simulink model "stm32eth"  (R2024a)
settings: Solver=FixedStepAuto  StartTime=0.0  StopTime=10  FixedStep=1/400  RelTol=1e-3  EnableMultiTasking=on
model workspace (MAT data in the model file):
  samp_time = 0.0025
libraries: stm32f4xxblockslib x6, spsTriangleGeneratorLib x1
settings Model: STM32="{\"DigitalPortWrite\":[{\"ID\":\"stm32eth:46\"},{\"ID\":\"stm32eth:45\"},{\"ID\":\"stm32eth:44\"},{\"ID\":\"stm32eth:43\"},{\"ID\":\"stm32eth:42\"},{\"ID\":\"stm32eth:41\"}]}"  Creator=Konstantin  LastModifiedBy=Konstantin
settings OptimizationCC: EnhancedBackFolding=on  PassReuseOutputArgsAs=Individual arguments  ZeroExternalMemoryAtStartup=off  ZeroInternalMemoryAtStartup=off  MaxStackSize=64  OptimizeBlockOrder=speed  DifferentSizesBufferReuse=on  OptimizationCustomize=off  EfficientTunableParamExpr=on
settings DebuggingCC: ParameterTunabilityLossMsg=error
settings HardwareCC: ProdBitPerPointer=32  ProdBitPerSizeT=32  ProdBitPerPtrDiffT=32  ProdLargestAtomicInteger=Long  ProdLargestAtomicFloat=Double  ProdWordSize=32  ProdLongLongMode=on  ProdHWDeviceType=ARM Compatible->ARM Cortex-M
settings SFSimCC: MATLABDynamicMemAlloc=off
settings RTWCC: Description=Embedded Coder  SystemTargetFile=ert.tlc  HardwareBoard=STM32G4xx Based  TemplateMakefile=ert_default_tmf  Toolchain=GNU Tools for ARM Embedded Processors
settings CodeAppCC: ForceParamTrailComments=on  IgnoreCustomStorageClasses=off  OperatorAnnotations=on  SimulinkDataObjDesc=on  SFDataObjDesc=on  InsertBlockDesc=on
settings ERTTargetCC: TargetLangStandard=C99 (ISO)  CodeReplacementLibrary=ARM Cortex-M  ExtModeTransport=3  ExtModeStaticAlloc=on  ExtModeStaticAllocSize=2048  ExtModeMexFile=ext_xcp  ExtModeIntrfLevel=Level2 - Open

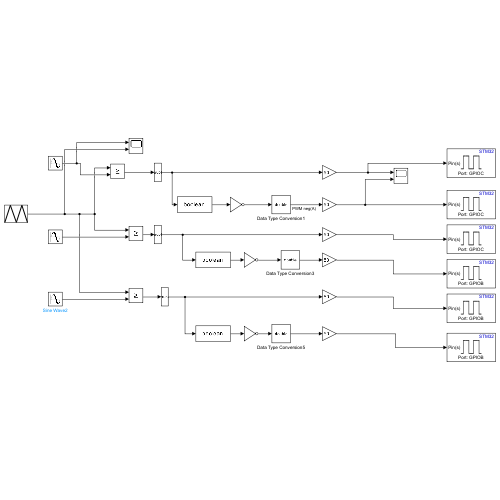
[thumbnail: Simulink's stored preview of the top-level diagram]
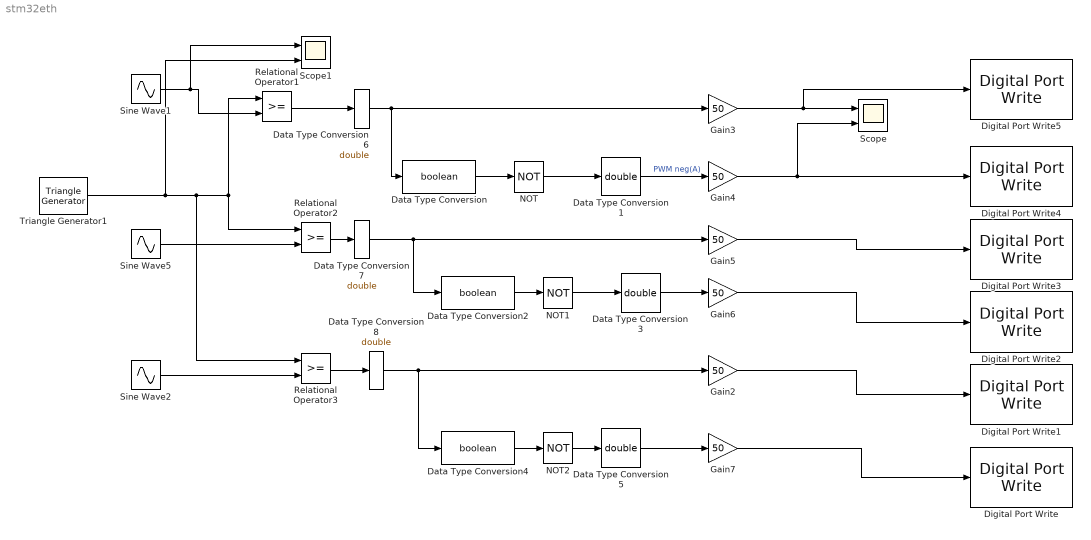
== system stm32eth ==
  Data Type Conversion : DataTypeConversion  OutDataTypeStr=boolean  SaturateOnIntegerOverflow=off  RndMeth=Floor
  Data Type Conversion1 : DataTypeConversion  OutDataTypeStr=double  RndMeth=Nearest  SaturateOnIntegerOverflow=off
  Data Type Conversion2 : DataTypeConversion  OutDataTypeStr=boolean  SaturateOnIntegerOverflow=off  RndMeth=Floor
  Data Type Conversion3 : DataTypeConversion  OutDataTypeStr=double  RndMeth=Nearest  SaturateOnIntegerOverflow=off
  Data Type Conversion4 : DataTypeConversion  OutDataTypeStr=boolean  SaturateOnIntegerOverflow=off  RndMeth=Floor
  Data Type Conversion5 : DataTypeConversion  OutDataTypeStr=double  RndMeth=Nearest  SaturateOnIntegerOverflow=off
  Data Type Conversion6 : DataTypeConversion  OutDataTypeStr=double  SaturateOnIntegerOverflow=off  RndMeth=Floor
  Data Type Conversion7 : DataTypeConversion  OutDataTypeStr=double  SaturateOnIntegerOverflow=off  RndMeth=Floor
  Data Type Conversion8 : DataTypeConversion  OutDataTypeStr=double  SaturateOnIntegerOverflow=off  RndMeth=Floor
  Digital Port Write : stm32f4xxblockslib/Digital Port Write  PortName=GPIOB  PinNumber=[5]  ReadOperation=off  IOAsArray=on  EnableSimPort=off  hoistedMaskSrc=ECSoC/ECSimCodegen/Digital Port Write
      settings: LibrarySourceBlock=stm32g4xxblockslib/Digital Port Write
  Digital Port Write1 : stm32f4xxblockslib/Digital Port Write  PortName=GPIOB  PinNumber=[4]  ReadOperation=off  IOAsArray=on  EnableSimPort=off  hoistedMaskSrc=ECSoC/ECSimCodegen/Digital Port Write
      settings: LibrarySourceBlock=stm32g4xxblockslib/Digital Port Write
  Digital Port Write2 : stm32f4xxblockslib/Digital Port Write  PortName=GPIOB  PinNumber=[3]  ReadOperation=off  IOAsArray=on  EnableSimPort=off  hoistedMaskSrc=ECSoC/ECSimCodegen/Digital Port Write
      settings: LibrarySourceBlock=stm32g4xxblockslib/Digital Port Write
  Digital Port Write3 : stm32f4xxblockslib/Digital Port Write  PortName=GPIOC  PinNumber=[3]  ReadOperation=off  IOAsArray=on  EnableSimPort=off  hoistedMaskSrc=ECSoC/ECSimCodegen/Digital Port Write
      settings: LibrarySourceBlock=stm32g4xxblockslib/Digital Port Write
  Digital Port Write4 : stm32f4xxblockslib/Digital Port Write  PortName=GPIOC  PinNumber=[2]  ReadOperation=off  IOAsArray=on  EnableSimPort=off  hoistedMaskSrc=ECSoC/ECSimCodegen/Digital Port Write
      settings: LibrarySourceBlock=stm32g4xxblockslib/Digital Port Write
  Digital Port Write5 : stm32f4xxblockslib/Digital Port Write  PortName=GPIOC  PinNumber=[1]  ReadOperation=off  IOAsArray=on  EnableSimPort=off  hoistedMaskSrc=ECSoC/ECSimCodegen/Digital Port Write
      settings: LibrarySourceBlock=stm32g4xxblockslib/Digital Port Write
  Gain{2..7} (6 alike) : Gain  Gain=50
  NOT : Logic  Operator=NOT  IconShape=distinctive  AllPortsSameDT=off  OutDataTypeStr=boolean
  NOT1 : Logic  Operator=NOT  IconShape=distinctive  AllPortsSameDT=off  OutDataTypeStr=boolean
  NOT2 : Logic  Operator=NOT  IconShape=distinctive  AllPortsSameDT=off  OutDataTypeStr=boolean
  Relational Operator1 : RelationalOperator  OutDataTypeStr=boolean  RndMeth=Simplest  InputSameDT=off
  Relational Operator2 : RelationalOperator  OutDataTypeStr=boolean  RndMeth=Simplest  InputSameDT=off
  Relational Operator3 : RelationalOperator  OutDataTypeStr=boolean  RndMeth=Simplest  InputSameDT=off
  Scope : Scope  NumInputPorts=2
  Scope1 : Scope  NumInputPorts=2
  Sine Wave1 : Sin  Frequency=0.050*2*pi  SampleTime=samp_time
  Sine Wave2 : Sin  Frequency=0.050*2*pi  Phase=4/3*pi  SampleTime=samp_time
  Sine Wave5 : Sin  Frequency=0.050*2*pi  Phase=2/3*pi  SampleTime=samp_time
  Triangle Generator1 : spsTriangleGeneratorLib/Triangle Generator  Freq=8  Phase=0  Ts=samp_time
  wires:
  Gain6/1 -> Digital Port Write2/1
  Gain5/1 -> Digital Port Write3/1
  Gain4/1 -> Scope/2, Digital Port Write4/1
  Data Type Conversion5/1 -> Gain7/1
  Data Type Conversion3/1 -> Gain6/1
  Data Type Conversion4/1 -> NOT2/1
  Data Type Conversion2/1 -> NOT1/1
  Data Type Conversion1/1 -> Gain4/1  "PWM neg(A)"
  NOT1/1 -> Data Type Conversion3/1
  NOT/1 -> Data Type Conversion1/1
  Data Type Conversion/1 -> NOT/1
  Gain7/1 -> Digital Port Write/1
  Gain2/1 -> Digital Port Write1/1
  NOT2/1 -> Data Type Conversion5/1
  Sine Wave1/1 -> Scope1/1, Relational Operator1/2
  Triangle Generator1/1 -> Scope1/2, Relational Operator3/1, Relational Operator1/1, Relational Operator2/1
  Sine Wave5/1 -> Relational Operator2/2
  Sine Wave2/1 -> Relational Operator3/2
  Relational Operator1/1 -> Data Type Conversion6/1
  Data Type Conversion6/1 -> Data Type Conversion/1, Gain3/1
  Relational Operator2/1 -> Data Type Conversion7/1
  Data Type Conversion7/1 -> Data Type Conversion2/1, Gain5/1
  Data Type Conversion8/1 -> Data Type Conversion4/1, Gain2/1
  Relational Operator3/1 -> Data Type Conversion8/1
  Gain3/1 -> Digital Port Write5/1, Scope/1
